simulink model "MADKAL"  (R2015a)
settings: Solver=ode45  StartTime=0.0  StopTime=10.0  RelTol=1e-3
values from neighbouring files (symbols this model uses):
  ba_e = zeros(3,1)    [Parameters.m]
  bb_e = 0    [Parameters.m]
  bg_e = zeros(3,1)    [Parameters.m]
  bm_e = zeros(3,1)    [Parameters.m]
  Ex = zeros(10,1)    [Parameters.m]
  g = 9.81    [Parameters.m]
  g_e = g    (= 9.81)    [Parameters.m]
  G_e = eye(3)    [Parameters.m]
  Ix_e = Ixx    (= 0.034736)    [Parameters.m]
  Iy_e = Iyy    (= 0.034736)    [Parameters.m]
  Iz_e = Izz    (= 0.069472)    [Parameters.m]
  kb_e = 1    [Parameters.m]
  m_e = m    (= 1.478)    [Parameters.m]
  Ma_e = eye(3)    [Parameters.m]
  mag_field = mag / norm(mag)    [Parameters.m]
  mf_e = mf_e /norm(mf_e)    [Parameters.m]
  Mg_e = eye(3)    [Parameters.m]
  P0 = 101325    [Parameters.m]
  P0_e = P0    (= 101325)    [Parameters.m]
  Q_e = 0.005*eye(10)    [Parameters.m]
  R_e = [ 0.0001   0 0 0 0 0 0 0 0 0 ... (first row only)    [Parameters.m]
  Ra = 286.9    [Parameters.m]
  Ra_e = Ra    (= 286.9)    [Parameters.m]
  T0 = 293.15    [Parameters.m]
  T0_e = T0    (= 293.15)    [Parameters.m]
  Ts = 1/200    (= 0.005)    [Parameters.m]
  Varx = 0.001*eye(10)    [Parameters.m]
undefined symbols (not defined in the file or in its folder): freqMadgwick, gain_aa, poles_aa, zeros_aa
libraries: Quadrotor_tools x16, simulink x1, simulink_extras x1
(part 2 of 2)

== matlab function MADKAL/Filtro di Kalman/Discrete EKF1/MATLAB Function ==
  data x_p settings: description=A-priori state estimate.
  data x settings: description=Corrected state estimate.
  data P_p settings: description=A-priori covariance estimate.
  data sensors settings: description=Measurements from the sensors.
  data U settings: description=Control signal (not needed at this step in the standard EKF implementation).
  data P settings: description=Corrected covariance estimate.
  data Ma_e settings: description=Axis misalignment and scaling matrix of the accelerometer.
  data ba_e settings: description=Bias of the accelerometer.
  data Mg_e settings: description=Axis misalignment and scaling matrix of the gyroscope.
  data bg_e settings: description=Bias of the gyroscope.
  data G_e settings: description=Axis misalignment and scaling matrix of the magnetometer (takes also accunt of the soft-iron distortions).
  data mf_e settings: description=Magnetic field measured in the earth frame.
  data bm_e settings: description=Bias of the magnetometer (takes also account of the hard-iron distortions).
  data kb_e settings: description=Scaling factor of the altimeter.
  data P0_e settings: description=Pressure measured at ground level.
  data g_e settings: description=Gravitational acceleration.
  data Ra_e settings: description=Gas constant of the air.
  data T0_e settings: description=Air temperature (K).
  data bb_e settings: description=Bias of the altimeter.
  data m_e settings: description=Mass of the quadrotor.
  data R_e settings: description=Covariance of the measurement noise.
  data: x_p input; x output; P_p input; sensors input; U input; P output; Ma_e parameter; ba_e parameter; Mg_e parameter; bg_e parameter; G_e parameter; mf_e parameter; bm_e parameter; kb_e parameter; P0_e parameter; g_e parameter; Ra_e parameter; T0_e parameter; bb_e parameter; m_e parameter; R_e parameter; K output
function [x, P, K] = EKF_update(x_p, P_p, sensors, U, Ma_e, ba_e, Mg_e, bg_e,...
    G_e, mf_e, bm_e, kb_e, P0_e, g_e, Ra_e, T0_e, bb_e, m_e, R_e)
%#codegen
% ----------------------------------------------------
% UPDATE STEP of the EKF
% ----------------------------------------------------

% ----------------------------------------------------
% State variables
% ----------------------------------------------------
% Linear velocity components
u = x_p(1);
v = x_p(2);
w = x_p(3);

% Angular velocity components
p = x_p(4);
q = x_p(5);
r = x_p(6);

% Angular position (Euler angles)
phi = x_p(7);
theta = x_p(8);
psi = x_p(9);

% Altitude
z = x_p(10);

% ----------------------------------------------------
% Rotation matrix
% ----------------------------------------------------
R = [cos(psi)*cos(theta), cos(psi)*sin(theta)*sin(phi)-sin(psi)*cos(phi),...
    cos(psi)*sin(theta)*cos(phi)+sin(psi)*sin(phi);
      sin(psi)*cos(theta), sin(psi)*sin(theta)*sin(phi)+cos(psi)*cos(phi),...
      sin(psi)*sin(theta)*cos(phi)-cos(psi)*sin(phi);
      -sin(theta) cos(theta)*sin(phi) cos(theta)*cos(phi)];

% ----------------------------------------------------
% Sensor equations
% ----------------------------------------------------
% Accelerometer
ya = Ma_e*[r*v - q*w; p*w - r*u; q*u - p*v + U(1)/m_e] + ba_e;

% Gyroscope
yg = Mg_e*[p; q; r] + bg_e;

% Magnetometer 
ym = G_e*R'*mf_e + bm_e;

% Altimeter (barometer)
yb = kb_e*P0_e*exp(-(g_e*z)/(Ra_e*T0_e)) + bb_e;


% ----------------------------------------------------
% Partial derivatives of the rotation matrix 
% with respect to phi, theta and psi.
% ----------------------------------------------------
Rdphi = [
    0, 0, 0;
    
    cos(psi)*sin(theta)*cos(phi) + sin(psi)*sin(phi),...
    sin(psi)*sin(theta)*cos(phi) - cos(psi)*sin(phi),...
    cos(theta)*cos(psi);
    
    -cos(psi)*sin(theta)*sin(phi) + sin(psi)*cos(phi),...
    -sin(psi)*sin(theta)*sin(phi) - cos(psi)*cos(phi),...
    -cos(theta)*sin(phi)
    ];

Rdtheta = [
    -cos(psi)*sin(theta),...
    -sin(psi)*sin(theta),...
    -cos(theta);
    
    cos(psi)*cos(theta)*sin(phi),...
    sin(psi)*cos(theta)*sin(phi),...
    -sin(theta)*sin(phi);
    
    cos(psi)*cos(theta)*cos(phi),...
    sin(psi)*cos(theta)*cos(phi),...
    -sin(theta)*cos(phi)
    ];

Rdpsi = [
    -sin(psi)*cos(theta), cos(psi)*cos(theta), 0;
    
    -sin(psi)*sin(theta)*sin(phi) - cos(psi)*cos(phi),...
    cos(psi)*sin(theta)*sin(phi) - sin(psi)*cos(phi),...
    0;
    
    -sin(psi)*sin(theta)*cos(phi) + cos(psi)*sin(phi),...
    cos(psi)*sin(theta)*cos(phi) + sin(psi)*sin(phi),...
    0
    ];

% ----------------------------------------------------
% Jacobian of the sensor equations.
% ----------------------------------------------------
% Accelerometer
J1 = Ma_e*[0 r -q; -r 0 p; q -p 0];
J2 = Ma_e*[0 -w v; w 0 -u; -v u 0];

% Magnetometer
J3 = [G_e*Rdphi*mf_e G_e*Rdtheta*mf_e G_e*Rdpsi*mf_e];

% Altimeter
Ja = -(kb_e*P0_e*g_e)/(Ra_e*T0_e)*exp(-(g_e*z)/(Ra_e*T0_e));

% Final matrix
 H = zeros(10);
 H(1:3,1:3) = J1;
 H(1:3,4:6) = J2;
 H(4:6,4:6) = Mg_e;
 H(7:9,7:9) = J3;
 H(10,10) = Ja;

% ----------------------------------------------------
% State update
% ----------------------------------------------------
% Measurement residual
y_res = sensors - [ya; yg; ym; yb];

% Innovation covariance
S = H*P_p*H' + R_e;

% Kalman gain
K = P_p*H'/S;

% Updated state estimate
x = x_p + K*y_res;

% Updated estimated covariance
P = (eye(10) - H*K)*P_p;

== matlab function MADKAL/Filtro di Kalman/Discrete EKF1/Predict  ==
  data x_old settings: description=State estimate at the previous step.
  data x_p settings: description=A-priori state estimate.
  data U_old settings: description=Control signal at the previous step.
  data P_p settings: description=A-priori covariance estimate.
  data P_old settings: description=Covariance estimate at the previous step.
  data Ix_e settings: description=X-axis component of the rotor intertia matrix.
  data Iy_e settings: description=Y-axis component of the rotor intertia matrix.
  data Iz_e settings: description=Z-axis component of the rotor intertia matrix.
  data g_e settings: description=Gravitational acceleration.
  data m_e settings: description=Mass of the quadrotor.
  data Ts settings: description=Sampling time.
  data Q_e settings: description=Covariance of the process noise (assumed constant).
  data: x_old input; x_p output; U_old input; P_p output; P_old input; Ix_e parameter; Iy_e parameter; Iz_e parameter; g_e parameter; m_e parameter; Ts parameter; Q_e parameter
function [x_p, P_p] = EKF_predict(x_old, U_old, P_old, Ix_e, Iy_e, Iz_e,...
                                    g_e, m_e, Ts, Q_e)
%#codegen
% ----------------------------------------------------
% PREDICTION STEP of the discrete time EKF
% ----------------------------------------------------

% ----------------------------------------------------
% State variables
% ----------------------------------------------------
% Linear velocity components
u_old = x_old(1);
v_old = x_old(2);
w_old = x_old(3);

% Angular velocity components
p_old = x_old(4);
q_old = x_old(5);
r_old = x_old(6);

% Angular position (Euler angles)
phi_old = x_old(7);
theta_old = x_old(8);

% Note: the state variables psi_old and z_old are not required
% in this step.

% ----------------------------------------------------
% State prediction
% ----------------------------------------------------
delta_x = zeros(10,1);

% State equations discretized using the forward Euler method.
delta_x(1) = r_old*v_old - q_old*w_old + g_e*sin(theta_old);
delta_x(2) = p_old*w_old - r_old*u_old - g_e*cos(theta_old)*sin(phi_old);
delta_x(3) = q_old*u_old - p_old*v_old - g_e*cos(theta_old)*cos(phi_old) +...
    U_old(1)/m_e;
delta_x(4) = (Iy_e - Iz_e)*q_old*r_old/Ix_e + U_old(2)/Ix_e;
delta_x(5) = (Iz_e - Ix_e)*p_old*r_old/Iy_e + U_old(3)/Iy_e;
delta_x(6) = (Ix_e - Iy_e)*p_old*q_old/Iz_e + U_old(4)/Iz_e;
delta_x(7) = p_old + sin(phi_old)*tan(theta_old)*q_old +...
    cos(phi_old)*tan(theta_old)*r_old;
delta_x(8) = cos(phi_old)*q_old - sin(phi_old)*r_old;
delta_x(9) = (sin(phi_old)*q_old)/cos(theta_old) +...
    (cos(phi_old)*r_old)/cos(theta_old);
delta_x(10) = -sin(theta_old)*u_old - cos(theta_old)*sin(phi_old)*v_old +...
    cos(theta_old)*cos(phi_old)*w_old;

x_p = x_old + Ts*delta_x;

% -----------------------------------------
% Covariance prediction
% -----------------------------------------
% Partial derivatives of the state equations.
F_old = eye(10);
F_old(1,2) = r_old;
F_old(1,3) = -q_old;
F_old(1,5) = -w_old;
F_old(1,6) = v_old;
F_old(1,8) = g_e*cos(theta_old);
F_old(2,1) = -r_old;
F_old(2,3) = p_old;
F_old(2,4) = w_old;
F_old(2,6) = -u_old;
F_old(2,7) = -g_e*cos(theta_old)*cos(phi_old);
F_old(2,8) = g_e*sin(theta_old)*sin(phi_old);
F_old(3,1) = q_old;
F_old(3,2) = -p_old;
F_old(3,4) = -v_old;
F_old(3,5) = u_old;
F_old(3,7) = g_e*cos(theta_old)*sin(phi_old);
F_old(3,8) = g_e*sin(theta_old)*cos(phi_old);
F_old(4,5) = (Iy_e - Iz_e)*r_old/Ix_e;
F_old(4,6) = (Iy_e - Iz_e)*q_old/Ix_e;
F_old(5,4) = (Iz_e - Ix_e)*r_old/Iy_e;
F_old(5,6) = (Iz_e - Ix_e)*p_old/Iy_e;
F_old(6,4) = (Ix_e - Iy_e)*q_old/Iz_e;
F_old(6,5) = (Ix_e - Iy_e)*p_old/Iz_e;
F_old(7,4) = 1;
F_old(7,5) = sin(phi_old)*tan(theta_old);
F_old(7,6) = cos(phi_old)*tan(theta_old);
F_old(7,7) = 1 + cos(phi_old)*tan(theta_old)*q_old - sin(phi_old)*cos(theta_old)*q_old;
F_old(7,8) = (sin(phi_old)*q_old + cos(phi_old)*r_old)/cos(theta_old)^2;
F_old(8,5) = cos(phi_old);
F_old(8,6) = -sin(phi_old);
F_old(8,7) = -cos(phi_old)*r_old - sin(phi_old)*q_old;
F_old(9,5) = sin(phi_old)/cos(theta_old);
F_old(9,6) = cos(phi_old)/cos(theta_old);
F_old(9,7) = (cos(phi_old)*q_old - sin(phi_old)*r_old)/cos(theta_old);
F_old(9,8) = sin(theta_old)*(sin(phi_old)*r_old + cos(phi_old)*q_old)/cos(theta_old)^2;
F_old(10,1) = -sin(theta_old);
F_old(10,2) = cos(theta_old)*sin(phi_old);
F_old(10,3) = cos(theta_old)*cos(phi_old);
F_old(10,7) = cos(theta_old)*cos(phi_old)*v_old - cos(theta_old)*sin(phi_old)*w_old;
F_old(10,8) = -cos(theta_old)*u_old - sin(theta_old)*sin(phi_old)*v_old -...
    cos(theta_old)*sin(theta_old)*w_old;

F_old = Ts*F_old;

% Covariance matrix update
P_p = F_old*P_old*F_old' + Q_e;
